simulink model "shoukongFDIA"  (R2024b)
settings: Solver=FixedStepDiscrete  StartTime=0.0  StopTime=10  FixedStep=1  RelTol=1e-3
settings Model: Creator=54238  LastModifiedBy=54238

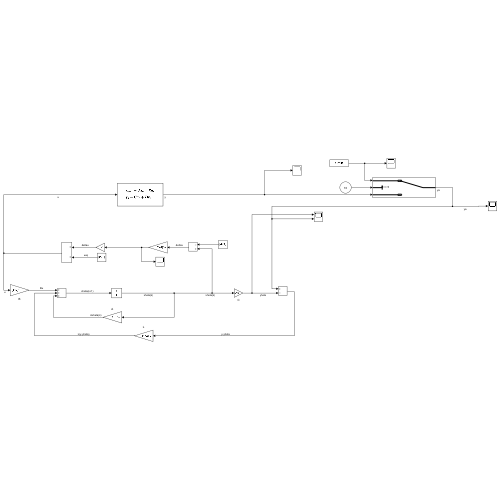
[thumbnail: Simulink's stored preview of the top-level diagram]
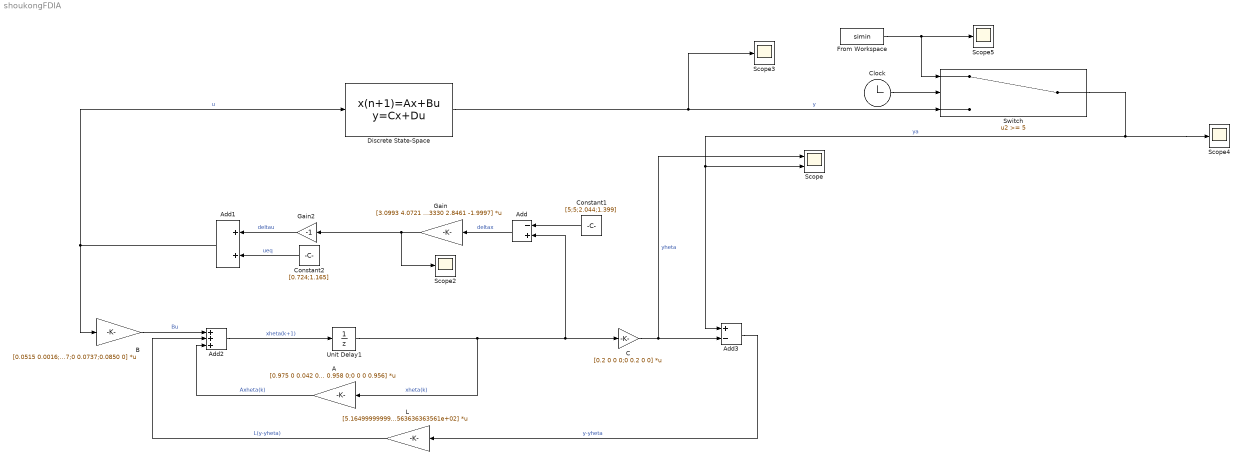
== system shoukongFDIA ==
  A : Gain  Gain=[0.975 0 0.042 0;0 0.977 0 0.044;0 0 0.958 0;0 0 0 0.956]  Multiplication=Matrix(K*u)
  Add : Sum  Inputs=-+
  Add1 : Sum
  Add2 : Sum  Inputs=+++
  Add3 : Sum  Inputs=+-
  B : Gain  Gain=[0.0515 0.0016;0.0019 0.0447;0 0.0737;0.0850 0]  Multiplication=Matrix(K*u)
  C : Gain  Gain=[0.2 0 0 0;0 0.2 0 0]  Multiplication=Matrix(K*u)
  Clock : Clock
  Constant1 : Constant  Value=[5;5;2.044;1.399]  VectorParams1D=off
  Constant2 : Constant  Value=[0.724;1.165]  VectorParams1D=off
  Discrete State-Space : DiscreteStateSpace  A=[0.975 0 0.042 0;0 0.977 0 0.044;0 0 0.958 0;0 0 0 0.956]  B=[0.0515 0.0016;0.0019 0.0447;0 0.0737;0.0850 0]  C=[0.2 0 0 0;0 0.2 0 0]  D=[0 0;0 0]  InitialCondition=[8 8 6 4]
  From Workspace : FromWorkspace  VariableName=simin
  Gain : Gain  Gain=[3.0993 4.0721 -2.0528 2.8417;3.9353 3.3330 2.8461 -1.9997]  Multiplication=Matrix(K*u)
  Gain2 : Gain  Gain=-1
  L : Gain  Gain=[5.164999999999978,0;0,14.164999999999758;30.424285714285460,0;0,2.243563636363561e+02]  Multiplication=Matrix(K*u)
  Scope : Scope  NumInputPorts=2
  Scope{2..5} (4 alike) : Scope
  Switch : Switch  Threshold=5  SaturateOnIntegerOverflow=off  InputSameDT=off
  Unit Delay1 : UnitDelay  SampleTime=-1  HasFrameUpgradeWarning=on
  wires:
  Unit Delay1/1 -> C/1, Add/2, A/1  "xheta(k)"
  Discrete State-Space/1 -> Scope3/1, Switch/3  "y"
  From Workspace/1 -> Scope5/1, Switch/1
  Clock/1 -> Switch/2
  Add2/1 -> Unit Delay1/1  "xheta(k+1)"
  Switch/1 -> Scope/2, Add3/1, Scope4/1  "ya"
  B/1 -> Add2/1  "Bu"
  A/1 -> Add2/3  "Axheta(k)"
  L/1 -> Add2/2  "L(y-yheta)"
  C/1 -> Scope/1, Add3/2  "yheta"
  Add/1 -> Gain/1  "deltax"
  Gain/1 -> Scope2/1, Gain2/1
  Add1/1 -> Discrete State-Space/1, B/1  "u"
  Gain2/1 -> Add1/1  "deltau"
  Constant1/1 -> Add/1
  Constant2/1 -> Add1/2  "ueq"
  Add3/1 -> L/1  "y-yheta"
